simulink model "iir2"  (Simulink 6.1)
settings: Solver=FixedStepDiscrete  StartTime=0.0  StopTime=10.0  RelTol=1e-3
libraries: dspsigops x7, simulink x1
settings Model: Creator=svenhoffmann  LastModifiedBy=svenhoffmann  ExtModeAutoUpdateStatusClock=off
settings DebuggingCC: SolverPrmCheckMsg=warning

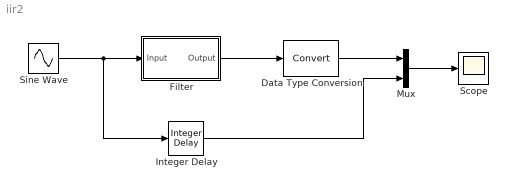
== system iir2 ==
  Data Type Conversion : DataTypeConversion
  Filter : Subsystem  Tag=FilterWizardSubSystem
  Integer Delay : simulink/Discrete/Integer Delay  vinit=0.0  samptime=-1  NumDelays=4
  Mux : Mux  Inputs=2
  Scope : Scope
  Sine Wave : Sin  Frequency=2*pi*100  SampleTime=1/1000
  wires:
  Sine Wave/1 -> Filter/1(Input), Integer Delay/1
  Filter/1(Output) -> Data Type Conversion/1
  Integer Delay/1 -> Mux/2
  Mux/1 -> Scope/1
  Data Type Conversion/1 -> Mux/1

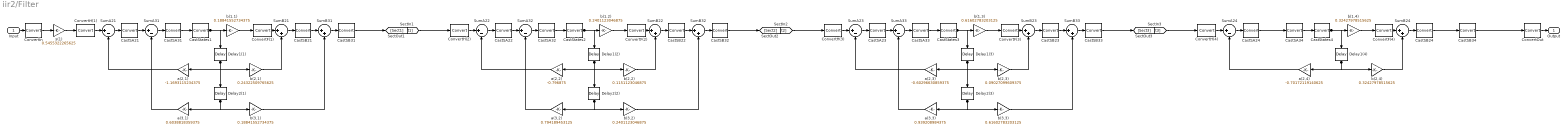
== system iir2/Filter ==
  Input : Inport  Port=1  LatchInput=off
  CastSA{21..24,31..34} (8 alike) : DataTypeConversion  OutDataTypeMode=Specify via dialog  OutDataType=sfix(40)  OutScaling=2^-26  RndMeth=Nearest  SaturateOnIntegerOverflow=on  LockScale=on
  CastSB{21..24,31..34} (8 alike) : DataTypeConversion  OutDataTypeMode=Specify via dialog  OutDataType=sfix(40)  OutScaling=2^-26  RndMeth=Nearest  SaturateOnIntegerOverflow=on  LockScale=on
  CastStates{1..4} (4 alike) : DataTypeConversion  OutDataTypeMode=Specify via dialog  OutScaling=2^-12  RndMeth=Nearest  SaturateOnIntegerOverflow=on  LockScale=on
  ConvertF(1) : DataTypeConversion  OutDataTypeMode=Specify via dialog  OutDataType=sfix(40)  OutScaling=2^-26  RndMeth=Nearest  SaturateOnIntegerOverflow=on  LockScale=on
  ConvertF(2) : DataTypeConversion  OutDataTypeMode=Specify via dialog  OutDataType=sfix(40)  OutScaling=2^-26  RndMeth=Nearest  SaturateOnIntegerOverflow=on  LockScale=on
  ConvertF(3) : DataTypeConversion  OutDataTypeMode=Specify via dialog  OutDataType=sfix(40)  OutScaling=2^-26  RndMeth=Nearest  SaturateOnIntegerOverflow=on  LockScale=on
  ConvertF(4) : DataTypeConversion  OutDataTypeMode=Specify via dialog  OutDataType=sfix(40)  OutScaling=2^-26  RndMeth=Nearest  SaturateOnIntegerOverflow=on  LockScale=on
  ConvertH(1) : DataTypeConversion  OutDataTypeMode=Specify via dialog  OutDataType=sfix(40)  OutScaling=2^-26  RndMeth=Nearest  SaturateOnIntegerOverflow=on  LockScale=on
  ConvertH(2) : DataTypeConversion  OutDataTypeMode=Specify via dialog  OutDataType=sfix(40)  OutScaling=2^-26  RndMeth=Nearest  SaturateOnIntegerOverflow=on  LockScale=on
  ConvertH(3) : DataTypeConversion  OutDataTypeMode=Specify via dialog  OutDataType=sfix(40)  OutScaling=2^-26  RndMeth=Nearest  SaturateOnIntegerOverflow=on  LockScale=on
  ConvertH(4) : DataTypeConversion  OutDataTypeMode=Specify via dialog  OutDataType=sfix(40)  OutScaling=2^-26  RndMeth=Nearest  SaturateOnIntegerOverflow=on  LockScale=on
  ConvertIn : DataTypeConversion  OutDataTypeMode=Specify via dialog  OutScaling=2^-14  RndMeth=Nearest  SaturateOnIntegerOverflow=on  LockScale=on
  ConvertOut : DataTypeConversion  OutDataTypeMode=Specify via dialog  OutScaling=2^-11  RndMeth=Nearest  SaturateOnIntegerOverflow=on  LockScale=on
  Delay1(1) : dspsigops/Delay  Orientation=down  dly_unit=Samples  delay=1  ic_detail=off  dif_ic_for_ch=off  dif_ic_for_dly=off  ic=0  reset_popup=None
  Delay1(2) : dspsigops/Delay  Orientation=down  dly_unit=Samples  delay=1  ic_detail=off  dif_ic_for_ch=off  dif_ic_for_dly=off  ic=0  reset_popup=None
  Delay1(3) : dspsigops/Delay  Orientation=down  dly_unit=Samples  delay=1  ic_detail=off  dif_ic_for_ch=off  dif_ic_for_dly=off  ic=0  reset_popup=None
  Delay1(4) : dspsigops/Delay  Orientation=down  dly_unit=Samples  delay=1  ic_detail=off  dif_ic_for_ch=off  dif_ic_for_dly=off  ic=0  reset_popup=None
  Delay2(1) : dspsigops/Delay  Orientation=down  dly_unit=Samples  delay=1  ic_detail=off  dif_ic_for_ch=off  dif_ic_for_dly=off  ic=0  reset_popup=None
  Delay2(2) : dspsigops/Delay  Orientation=down  dly_unit=Samples  delay=1  ic_detail=off  dif_ic_for_ch=off  dif_ic_for_dly=off  ic=0  reset_popup=None
  Delay2(3) : dspsigops/Delay  Orientation=down  dly_unit=Samples  delay=1  ic_detail=off  dif_ic_for_ch=off  dif_ic_for_dly=off  ic=0  reset_popup=None
  SumA{21..24,31..33} (7 alike) : Sum  Inputs=|+-  OutDataTypeMode=Specify via dialog  OutDataType=sfix(34)  OutScaling=2^-26  RndMeth=Nearest  SaturateOnIntegerOverflow=on  LockScale=on
  SumB{21..24,31..33} (7 alike) : Sum  Inputs=|++  OutDataTypeMode=Specify via dialog  OutDataType=sfix(34)  OutScaling=2^-26  RndMeth=Nearest  SaturateOnIntegerOverflow=on  LockScale=on
  a(2,1) : Gain  Orientation=left  Gain=-1.1693115234375  ParameterDataTypeMode=Specify via dialog  ParameterScalingMode=Use specified scaling  ParameterScaling=2^-14  OutDataTypeMode=Specify via dialog  OutDataType=sfix(32)  OutScaling=2^-26  RndMeth=Nearest  SaturateOnIntegerOverflow=on  LockScale=on
  a(2,2) : Gain  Orientation=left  Gain=-0.796875  ParameterDataTypeMode=Specify via dialog  ParameterScalingMode=Use specified scaling  ParameterScaling=2^-14  OutDataTypeMode=Specify via dialog  OutDataType=sfix(32)  OutScaling=2^-26  RndMeth=Nearest  SaturateOnIntegerOverflow=on  LockScale=on
  a(2,3) : Gain  Orientation=left  Gain=-0.60296630859375  ParameterDataTypeMode=Specify via dialog  ParameterScalingMode=Use specified scaling  ParameterScaling=2^-14  OutDataTypeMode=Specify via dialog  OutDataType=sfix(32)  OutScaling=2^-26  RndMeth=Nearest  SaturateOnIntegerOverflow=on  LockScale=on
  a(2,4) : Gain  Orientation=left  Gain=-0.70172119140625  ParameterDataTypeMode=Specify via dialog  ParameterScalingMode=Use specified scaling  ParameterScaling=2^-14  OutDataTypeMode=Specify via dialog  OutDataType=sfix(32)  OutScaling=2^-26  RndMeth=Nearest  SaturateOnIntegerOverflow=on  LockScale=on
  a(3,1) : Gain  Orientation=left  Gain=0.6038818359375  ParameterDataTypeMode=Specify via dialog  ParameterScalingMode=Use specified scaling  ParameterScaling=2^-14  OutDataTypeMode=Specify via dialog  OutDataType=sfix(32)  OutScaling=2^-26  RndMeth=Nearest  SaturateOnIntegerOverflow=on  LockScale=on
  a(3,2) : Gain  Orientation=left  Gain=0.794189453125  ParameterDataTypeMode=Specify via dialog  ParameterScalingMode=Use specified scaling  ParameterScaling=2^-14  OutDataTypeMode=Specify via dialog  OutDataType=sfix(32)  OutScaling=2^-26  RndMeth=Nearest  SaturateOnIntegerOverflow=on  LockScale=on
  a(3,3) : Gain  Orientation=left  Gain=0.939208984375  ParameterDataTypeMode=Specify via dialog  ParameterScalingMode=Use specified scaling  ParameterScaling=2^-14  OutDataTypeMode=Specify via dialog  OutDataType=sfix(32)  OutScaling=2^-26  RndMeth=Nearest  SaturateOnIntegerOverflow=on  LockScale=on
  b(1,1) : Gain  Gain=0.18841552734375  ParameterDataTypeMode=Specify via dialog  ParameterScalingMode=Use specified scaling  ParameterScaling=2^-14  OutDataTypeMode=Specify via dialog  OutDataType=sfix(32)  OutScaling=2^-26  RndMeth=Nearest  SaturateOnIntegerOverflow=on  LockScale=on
  b(1,2) : Gain  Gain=0.2401123046875  ParameterDataTypeMode=Specify via dialog  ParameterScalingMode=Use specified scaling  ParameterScaling=2^-14  OutDataTypeMode=Specify via dialog  OutDataType=sfix(32)  OutScaling=2^-26  RndMeth=Nearest  SaturateOnIntegerOverflow=on  LockScale=on
  b(1,3) : Gain  Gain=0.61602783203125  ParameterDataTypeMode=Specify via dialog  ParameterScalingMode=Use specified scaling  ParameterScaling=2^-14  OutDataTypeMode=Specify via dialog  OutDataType=sfix(32)  OutScaling=2^-26  RndMeth=Nearest  SaturateOnIntegerOverflow=on  LockScale=on
  b(1,4) : Gain  Gain=0.32427978515625  ParameterDataTypeMode=Specify via dialog  ParameterScalingMode=Use specified scaling  ParameterScaling=2^-14  OutDataTypeMode=Specify via dialog  OutDataType=sfix(32)  OutScaling=2^-26  RndMeth=Nearest  SaturateOnIntegerOverflow=on  LockScale=on
  b(2,1) : Gain  Gain=0.24322509765625  ParameterDataTypeMode=Specify via dialog  ParameterScalingMode=Use specified scaling  ParameterScaling=2^-14  OutDataTypeMode=Specify via dialog  OutDataType=sfix(32)  OutScaling=2^-26  RndMeth=Nearest  SaturateOnIntegerOverflow=on  LockScale=on
  b(2,2) : Gain  Gain=0.1151123046875  ParameterDataTypeMode=Specify via dialog  ParameterScalingMode=Use specified scaling  ParameterScaling=2^-14  OutDataTypeMode=Specify via dialog  OutDataType=sfix(32)  OutScaling=2^-26  RndMeth=Nearest  SaturateOnIntegerOverflow=on  LockScale=on
  b(2,3) : Gain  Gain=0.09027099609375  ParameterDataTypeMode=Specify via dialog  ParameterScalingMode=Use specified scaling  ParameterScaling=2^-14  OutDataTypeMode=Specify via dialog  OutDataType=sfix(32)  OutScaling=2^-26  RndMeth=Nearest  SaturateOnIntegerOverflow=on  LockScale=on
  b(2,4) : Gain  Gain=0.32427978515625  ParameterDataTypeMode=Specify via dialog  ParameterScalingMode=Use specified scaling  ParameterScaling=2^-14  OutDataTypeMode=Specify via dialog  OutDataType=sfix(32)  OutScaling=2^-26  RndMeth=Nearest  SaturateOnIntegerOverflow=on  LockScale=on
  b(3,1) : Gain  Gain=0.18841552734375  ParameterDataTypeMode=Specify via dialog  ParameterScalingMode=Use specified scaling  ParameterScaling=2^-14  OutDataTypeMode=Specify via dialog  OutDataType=sfix(32)  OutScaling=2^-26  RndMeth=Nearest  SaturateOnIntegerOverflow=on  LockScale=on
  b(3,2) : Gain  Gain=0.2401123046875  ParameterDataTypeMode=Specify via dialog  ParameterScalingMode=Use specified scaling  ParameterScaling=2^-14  OutDataTypeMode=Specify via dialog  OutDataType=sfix(32)  OutScaling=2^-26  RndMeth=Nearest  SaturateOnIntegerOverflow=on  LockScale=on
  b(3,3) : Gain  Gain=0.61602783203125  ParameterDataTypeMode=Specify via dialog  ParameterScalingMode=Use specified scaling  ParameterScaling=2^-14  OutDataTypeMode=Specify via dialog  OutDataType=sfix(32)  OutScaling=2^-26  RndMeth=Nearest  SaturateOnIntegerOverflow=on  LockScale=on
  s(1) : Gain  Gain=0.5455322265625  ParameterDataTypeMode=Specify via dialog  ParameterScalingMode=Use specified scaling  ParameterScaling=2^-14  OutDataTypeMode=Specify via dialog  OutScaling=2^-9  RndMeth=Nearest  SaturateOnIntegerOverflow=on  LockScale=on
  Output : Outport
  wires:
  Input/1 -> ConvertIn/1
  ConvertIn/1 -> s(1)/1
  s(1)/1 -> ConvertH(1)/1
  ConvertH(1)/1 -> SumA21/1
  SumA21/1 -> CastSA21/1
  CastSA21/1 -> SumA31/1
  SumA31/1 -> CastSA31/1
  CastSA31/1 -> CastStates1/1
  CastStates1/1 -> b(1,1)/1, Delay1(1)/1
  b(1,1)/1 -> ConvertF(1)/1
  ConvertF(1)/1 -> SumB21/1
  SumB21/1 -> CastSB21/1
  CastSB21/1 -> SumB31/1
  SumB31/1 -> CastSB31/1
  CastSB31/1 -> [Sect1]
  Delay1(1)/1 -> Delay2(1)/1, b(2,1)/1, a(2,1)/1
  b(2,1)/1 -> SumB21/2
  Delay2(1)/1 -> b(3,1)/1, a(3,1)/1
  b(3,1)/1 -> SumB31/2
  a(2,1)/1 -> SumA21/2
  a(3,1)/1 -> SumA31/2
  [Sect1] -> ConvertH(2)/1
  ConvertH(2)/1 -> SumA22/1
  SumA22/1 -> CastSA22/1
  CastSA22/1 -> SumA32/1
  SumA32/1 -> CastSA32/1
  CastSA32/1 -> CastStates2/1
  CastStates2/1 -> b(1,2)/1, Delay1(2)/1
  b(1,2)/1 -> ConvertF(2)/1
  ConvertF(2)/1 -> SumB22/1
  SumB22/1 -> CastSB22/1
  CastSB22/1 -> SumB32/1
  SumB32/1 -> CastSB32/1
  CastSB32/1 -> [Sect2]
  Delay1(2)/1 -> Delay2(2)/1, b(2,2)/1, a(2,2)/1
  b(2,2)/1 -> SumB22/2
  Delay2(2)/1 -> b(3,2)/1, a(3,2)/1
  b(3,2)/1 -> SumB32/2
  a(2,2)/1 -> SumA22/2
  a(3,2)/1 -> SumA32/2
  [Sect2] -> ConvertH(3)/1
  ConvertH(3)/1 -> SumA23/1
  SumA23/1 -> CastSA23/1
  CastSA23/1 -> SumA33/1
  SumA33/1 -> CastSA33/1
  CastSA33/1 -> CastStates3/1
  CastStates3/1 -> b(1,3)/1, Delay1(3)/1
  b(1,3)/1 -> ConvertF(3)/1
  ConvertF(3)/1 -> SumB23/1
  SumB23/1 -> CastSB23/1
  CastSB23/1 -> SumB33/1
  SumB33/1 -> CastSB33/1
  CastSB33/1 -> [Sect3]
  Delay1(3)/1 -> Delay2(3)/1, b(2,3)/1, a(2,3)/1
  b(2,3)/1 -> SumB23/2
  Delay2(3)/1 -> b(3,3)/1, a(3,3)/1
  b(3,3)/1 -> SumB33/2
  a(2,3)/1 -> SumA23/2
  a(3,3)/1 -> SumA33/2
  [Sect3] -> ConvertH(4)/1
  ConvertH(4)/1 -> SumA24/1
  SumA24/1 -> CastSA24/1
  CastSA34/1 -> CastStates4/1
  CastStates4/1 -> b(1,4)/1, Delay1(4)/1
  b(1,4)/1 -> ConvertF(4)/1
  ConvertF(4)/1 -> SumB24/1
  SumB24/1 -> CastSB24/1
  ConvertOut/1 -> Output/1
  CastSB34/1 -> ConvertOut/1
  Delay1(4)/1 -> b(2,4)/1, a(2,4)/1
  b(2,4)/1 -> SumB24/2
  a(2,4)/1 -> SumA24/2
  CastSB24/1 -> CastSB34/1
  CastSA24/1 -> CastSA34/1
